simulink model "hw6Q1_model"  (R2021a)
settings: Solver=VariableStepAuto  StartTime=0.0  StopTime=time_end  RelTol=1e-3
values from neighbouring files (symbols this model uses):
  K_i = K_i_list(i)    [hw6Q1.m]    (also in hw6Q2.m = K_i_list(ii); hw6Q2_tony.m = K_i_list(kk); hw6Q3.m = 0.5)
  K_p = 1    [hw6Q1.m]    (also in hw6Q2.m = K_p_list(pp); hw6Q2_tony.m = K_p_list(kk); hw6Q3.m)
  T_L_a = 0.0    (= 0)    [hw6Q1.m]
settings Model: Creator=kaiyu  LastModifiedBy=kaiyu

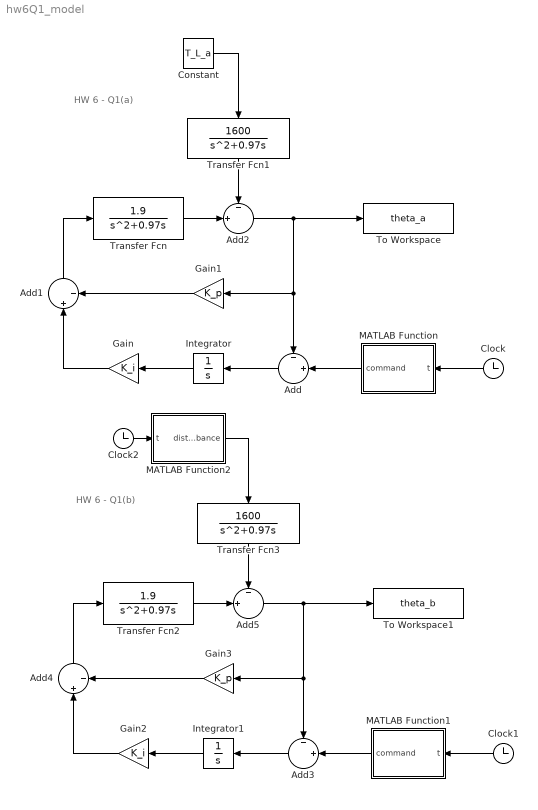
== system hw6Q1_model ==
  note: HW 6 - Q1(a)
  note: HW 6 - Q1(b)
  Add{,2..3,5} (4 alike) : Sum  Inputs=-|+||
  Add1 : Sum  Inputs=||+|-
  Add4 : Sum  Inputs=||+|-
  Clock : Clock
  Clock1 : Clock
  Clock2 : Clock
  Constant : Constant  Value=T_L_a
  Gain : Gain  Gain=K_i
  Gain1 : Gain  Gain=K_p
  Gain2 : Gain  Gain=K_i
  Gain3 : Gain  Gain=K_p
  Integrator : Integrator
  Integrator1 : Integrator
  MATLAB Function : MATLAB Function  TreatAsAtomicUnit=on
  MATLAB Function1 : MATLAB Function  TreatAsAtomicUnit=on
  MATLAB Function2 : MATLAB Function  TreatAsAtomicUnit=on
  To Workspace : ToWorkspace  VariableName=theta_a  SaveFormat=Timeseries  SampleTime=-1
  To Workspace1 : ToWorkspace  VariableName=theta_b  SaveFormat=Timeseries  SampleTime=-1
  Transfer Fcn : TransferFcn  Numerator=[1.9]  Denominator=[1 0.97 0]
  Transfer Fcn1 : TransferFcn  Numerator=[1600]  Denominator=[1 0.97 0]
  Transfer Fcn2 : TransferFcn  Numerator=[1.9]  Denominator=[1 0.97 0]
  Transfer Fcn3 : TransferFcn  Numerator=[1600]  Denominator=[1 0.97 0]
  wires:
  MATLAB Function/1(command) -> Add/2
  Add/1 -> Integrator/1
  Integrator/1 -> Gain/1
  Gain/1 -> Add1/1
  Gain1/1 -> Add1/2
  Add1/1 -> Transfer Fcn/1
  Transfer Fcn/1 -> Add2/2
  Transfer Fcn1/1 -> Add2/1
  Constant/1 -> Transfer Fcn1/1
  Add2/1 -> Gain1/1, Add/1, To Workspace/1
  Clock/1 -> MATLAB Function/1(t)
  MATLAB Function1/1(command) -> Add3/2
  Gain3/1 -> Add4/2
  Add4/1 -> Transfer Fcn2/1
  Clock1/1 -> MATLAB Function1/1(t)
  Gain2/1 -> Add4/1
  MATLAB Function2/1(disturbance) -> Transfer Fcn3/1
  Integrator1/1 -> Gain2/1
  Transfer Fcn3/1 -> Add5/1
  Transfer Fcn2/1 -> Add5/2
  Add3/1 -> Integrator1/1
  Add5/1 -> Gain3/1, Add3/1, To Workspace1/1
  Clock2/1 -> MATLAB Function2/1(t)

== matlab function hw6Q1_model/MATLAB Function ==
  data: t input; command output
function command = reference(t)
if (0 <= t) && (t <= 2)
    r = 0;
else
    r = 0.5;
end
command = r;

== matlab function hw6Q1_model/MATLAB Function2 ==
  data: t input; disturbance output
function disturbance = T_L_b(t)
if (t < 6)
    d = 0;
else
    d = 0.0003;
end    
disturbance = d;

== matlab function hw6Q1_model/MATLAB Function1 ==
  data: t input; command output
function command = reference(t)
if (0 <= t) && (t <= 2)
    r = 0;
else
    r = 0.5;
end
command = r;
